simulink model "model"  (R2023a)
settings: Solver=VariableStepAuto  StartTime=0.0  StopTime=10.0  RelTol=1e-3
settings Model: Creator=30296  LastModifiedBy=30296

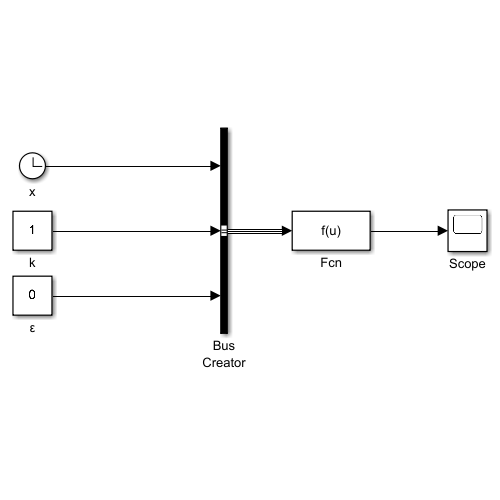
[thumbnail: Simulink's stored preview of the top-level diagram]
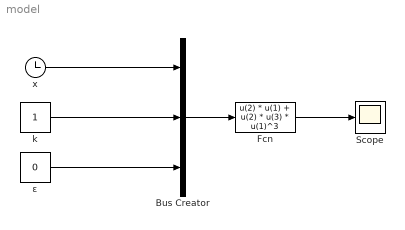
== system model ==
  Bus Creator : BusCreator  Inputs=3
  Fcn : Fcn  Expr=u(2) * u(1) + u(2) * u(3) * u(1)^3
  Scope : Scope
  k : Constant
  x : Clock
  ε : Constant  Value=0
  wires:
  k/1 -> Bus Creator/2
  ε/1 -> Bus Creator/3
  x/1 -> Bus Creator/1
  Bus Creator/1 -> Fcn/1
  Fcn/1 -> Scope/1
